simulink model "mppt"  (R2022b)
settings: Solver=ode23tb  StartTime=0.0  StopTime=5  RelTol=1e-3
libraries: spsSeriesRLCBranchLib x4, spsCurrentMeasurementLib x1, spsDiodeLib x1, spsIGBTLib x1, spsPVArrayLib x1, spsPWMGeneratorDCDCLib x1, spsVoltageMeasurementLib x1, sps_lib x1
settings Model: Creator=Flavia Saldanha  LastModifiedBy=Flavia Saldanha
settings DataIOCC: ExternalInput=irradiance, temperature  SaveFormat=Array

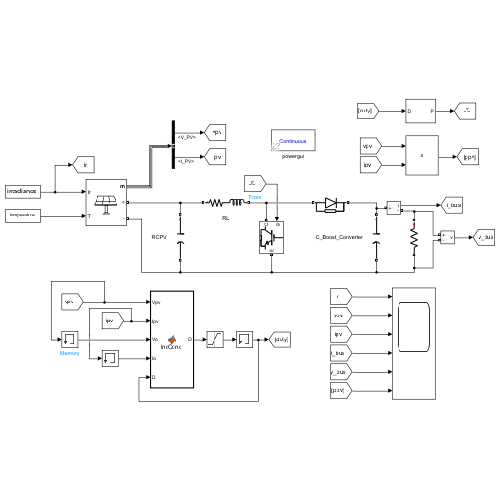
[thumbnail: Simulink's stored preview of the top-level diagram]
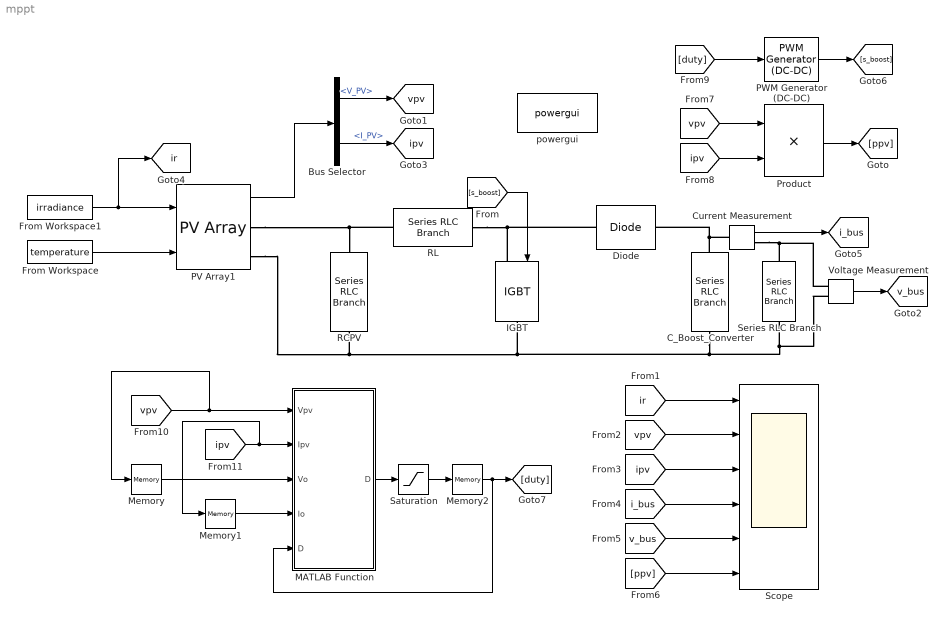
== system mppt ==
  Bus Selector : BusSelector  OutputSignals=V_PV,I_PV
  C_Boost_Converter : spsSeriesRLCBranchLib/Series RLC Branch  LConnTagsString=__new0  RConnTagsString=__new0  BranchType=C  Resistance=1e-4  Inductance=1e-3  SetiL0=off  InitialCurrent=0  Capacitance=0.05  Setx0=off  InitialVoltage=0  Measurements=None
  Current Measurement : spsCurrentMeasurementLib/Current Measurement  PhasorSimulation=off  OutputType=Complex  PSBequivalent=0
  Diode : spsDiodeLib/Diode  Ron=0.001  Lon=0  Vf=0.8  IC=0  UseSnubber=0  Rs=500  Cs=250e-9  Measurements=off
  From Workspace : FromWorkspace  VariableName=temperature
  From Workspace1 : FromWorkspace  VariableName=irradiance
  IGBT : spsIGBTLib/IGBT  Ron=0.001  Lon=0  Vf=1  Tf=1e-6  Tt=2e-6  IC=0  Rs=1e5  Cs=inf  Measurements=off
  MATLAB Function : MATLAB Function  TreatAsAtomicUnit=on
  Memory : Memory
  Memory1 : Memory
  Memory2 : Memory
  PV Array1 : spsPVArrayLib/PV Array  Npar=12  Nser=4  PlotType=array @ 1000 W/m2 & specified temperatures  S_vec="[ 1000  500  100 ]"  Temp_C_vec="[ 45 25  ]"  ModuleName=User-defined  PlotWhenSelected=off  Pm=213.15  Ncell=60  Voc=36.3  Isc=7.84  Vm=29  Im=7.35  beta_Voc_pc=-0.36099  alpha_Isc_pc=0.102  beta_Voc=-0.13104  alpha_Isc=0.0079968  IL=7.8654  I0=2.9273e-10  nI=0.98119  Rsh=313.0553  Rs=0.39381  RobustModel=off  RobustCellTemperature=313.3991  BAL=on  Tc=1e-6  Tfilter=5e-5
  PWM Generator (DC-DC) : spsPWMGeneratorDCDCLib/PWM Generator (DC-DC)  Fsw=5000  Ts=10e-6
  Product : Product
  RCPV : spsSeriesRLCBranchLib/Series RLC Branch  LConnTagsString=__new0  RConnTagsString=__new0  BranchType=C  Resistance=100e-6  Inductance=1e-3  SetiL0=off  InitialCurrent=0  Capacitance=100e-6  Setx0=off  InitialVoltage=0  Measurements=None
  RL : spsSeriesRLCBranchLib/Series RLC Branch  LConnTagsString=__new0  RConnTagsString=__new0  BranchType=RL  Resistance=1e-3  Inductance=0.01  SetiL0=off  InitialCurrent=0  Capacitance=100e-6  Setx0=off  InitialVoltage=0  Measurements=None
  Saturation : Saturate  UpperLimit=0.9  LowerLimit=0
  Scope : Scope  NumInputPorts=6
  Series RLC Branch : spsSeriesRLCBranchLib/Series RLC Branch  LConnTagsString=__new0  RConnTagsString=__new0  BranchType=R  Resistance=40  Inductance=1e-3  SetiL0=off  InitialCurrent=0  Capacitance=1e-6  Setx0=off  InitialVoltage=0  Measurements=None
  Voltage Measurement : spsVoltageMeasurementLib/Voltage Measurement  PhasorSimulation=off  OutputType=Complex  PSBequivalent=0
  powergui : sps_lib/powergui  Priority=1  SimulationMode=Continuous  SampleTime=1e-6  frequency=60  Iterations=50  frequencyindice=0  Pbase=100e6  ErrMax=1e-4  UnitsV=kV  UnitsW=MW  buscounter=0  FunctionMessages=off  echomessages=off  EnableUseOfTLC=off  CurrentSourceSwitches=off  DisableSnubberDevices=off  DisableRonSwitches=off  DisableVfSwitches=off  DisplayEquations=off  AutomaticDiscreteSolvers=off  SolverType=Tustin/Backward Euler (TBE)  Interpol=off  ExternalGateDelay=off  methode=off  Ts=100  x0status=blocks  SPID=on  SwTol=0  HookPort=off  NonlinearTolerance=1e-4  nMaxIteration=100  ContinueOnMaxIteration=off  RestoreLinks=warning  ResistiveCurrentMeasurement=off  Frange=[0:2:500]  Ylog=off  Xlog=on  ShowGrid=off  save=off  variable=ZData  structure=0  ZoomFFT=off  StartTime=0.0  cycles=1  DisplayStyle=1  fundamental=60  FreqAxis=off  MaxFrequency=1000  frequencyindicesteady=1  RmsSteady=1  display=off
  tag scope: i_bus=global, ipv=global, ir=global, v_bus=global, vpv=global
  wires:
  PV Array1/1 -> Bus Selector/1
  Bus Selector/1 -> [vpv]  "<V_PV>"
  Bus Selector/2 -> [ipv]  "<I_PV>"
  [s_boost] -> IGBT/1
  Voltage Measurement/1 -> [v_bus]
  Current Measurement/1 -> [i_bus]
  [ir] -> Scope/1
  [vpv] -> Scope/2
  [ipv] -> Scope/3
  [i_bus] -> Scope/4
  [v_bus] -> Scope/5
  [ppv] -> Scope/6
  Product/1 -> [ppv]
  [vpv] -> Product/1
  [ipv] -> Product/2
  PWM Generator (DC-DC)/1 -> [s_boost]
  [duty] -> PWM Generator (DC-DC)/1
  [vpv] -> Memory/1, MATLAB Function/1(Vpv)
  Memory/1 -> MATLAB Function/3(Vo)
  Memory1/1 -> MATLAB Function/4(Io)
  [ipv] -> Memory1/1, MATLAB Function/2(Ipv)
  MATLAB Function/1(D) -> Saturation/1
  Saturation/1 -> Memory2/1
  Memory2/1 -> MATLAB Function/5("D "), [duty]
  From Workspace1/1 -> [ir], PV Array1/1
  From Workspace/1 -> PV Array1/2
  connections:
  Series RLC Branch/RConn1 -- Voltage Measurement/LConn2 -- C_Boost_Converter/RConn1 -- PV Array1/RConn2 -- RCPV/RConn1 -- IGBT/RConn1
  RL/RConn1 -- IGBT/LConn1 -- Diode/LConn1
  Current Measurement/RConn1 -- Series RLC Branch/LConn1 -- Voltage Measurement/LConn1
  Current Measurement/LConn1 -- C_Boost_Converter/LConn1 -- Diode/RConn1
  PV Array1/RConn1 -- RL/LConn1 -- RCPV/LConn1

== matlab function mppt/MATLAB Function ==
  data: Vpv input; D output; Ipv input; Vo input; Io input; D input
function D = IncCond(Vpv, Ipv, Vo, Io, D)

dv=Vpv-Vo;
di=Ipv-Io;
d=0.00005;

if dv == 0
    if di == 0
        m=D;
    else
        m=D+d;
    end
else
    if di/dv == -Ipv/Vpv
        m=D;
    else 
        if di/dv > -Ipv/Vpv
            m=D-d;
        else
            m=D+d;
        end
    end

end
D=m;
end
